simulink model "awe_mpc_sim"  (R2017b)
settings: Solver=ode1  StartTime=0.0  StopTime=10.0  FixedStep=0.1  RelTol=1e-3
settings Model: Creator=itz  LastModifiedBy=itz

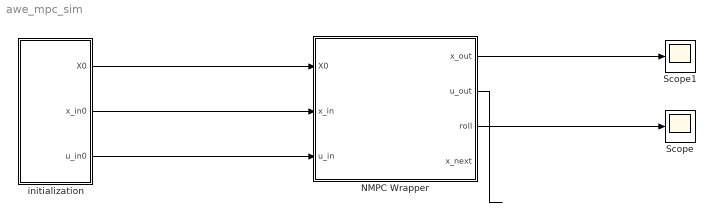
== system awe_mpc_sim ==
  NMPC Wrapper : MATLAB Function  TreatAsAtomicUnit=on
  Scope : Scope
  Scope1 : Scope
  initialization : MATLAB Function  TreatAsAtomicUnit=on
  wires:
  NMPC Wrapper/1(x_out) -> Scope1/1
  NMPC Wrapper/2(u_out) -> ?
  initialization/1(X0) -> NMPC Wrapper/1(X0)
  NMPC Wrapper/3(roll) -> Scope/1
  initialization/2(x_in0) -> NMPC Wrapper/2(x_in)
  initialization/3(u_in0) -> NMPC Wrapper/3(u_in)

== matlab function awe_mpc_sim/initialization ==
  data: X0 output; x_in0 output; u_in0 output
function [X0,x_in0,u_in0] = fcn()

vw = -5;
r = 220;
circle_azimut = -pi/2;
circle_elevation = 20/180*pi;
R = atan(90/220);%25/180*pi;% Reference opening angle of the circle
init = 1;

N=30;

X0 = [-pi/2 ,R+circle_elevation ,-pi/2 ,0.0, 50 ];

x_in0 = repmat(X0,N+1,1);

u_in0 = zeros(N,1);

end

== matlab function awe_mpc_sim/NMPC Wrapper ==
  data: X0 input; x_out output; x_in input; u_in input; u_out output; roll output; x_next output
function [x_out,u_out,roll,x_next] = fcn(X0,x_in,u_in)


% OnlineData (Parameters)
vw = -5;
r = 220;
circle_azimut = -pi/2;
circle_elevation = 20/180*pi;
R = atan(90/220);%25/180*pi;% Reference opening angle of the circle
init = 1;

N=30;

% If its the very first step these are empty, thus need to be initialized
if isempty(X0)
    X0 = [-pi/2 ,R+circle_elevation ,-pi/2 ,0.0, 50 ];
end
if isempty(x_in)
    x_in = repmat(X0,N+1,1);
end
if isempty(u_in)
    u_in = zeros(N,1);
end

    


% Propagate Horizon
x_in(1:end-1,:) = x_in(2:end,:);
x_in(end,:) = x_in(end,:);
u_in(1:end-1,:) = u_in(2:end,:);
u_in(end,:) = u_in(end,:);




%% Prepare Simulation
% Fill input vector
input.x0 = X0;
input.x = x_in;
input.od = repmat([vw,r,circle_azimut,circle_elevation,init],N+1,1);

Uref = zeros(N,1);
input.u = u_in;

Yref = ones(N,1)*[R,1];

input.y = [ Yref, Uref];
input.yN = [R,1];

input.W = diag([1 0 0.01]);
input.WN = diag([1 0]);

output.info.status = 0;  % This had to be moved before .x and .u
output.info.cpuTime = 0;  % such that the field are in correct order
output.info.kktValue = 0;  % otherwise it does not work...
output.info.objValue = 0;
output.info.nIterations = 0;
output.x=input.x;  % This is just to define output array size
output.u=input.u;  % Without this simulink has issues to figure out port sizes

coder.extrinsic('awe_MPCstep');  % This is to tell Simulink compiler not to try to compile the solver again
output = awe_MPCstep(input); % Solve NMPC





x_out = output.x;
u_out = output.u;
roll  = output.x(1,4); % Current Roll Command
x_next = output.x(2,:);
